simulink model "schemat_macierze"  (R2015a)
settings: Solver=ode45  StartTime=0.0  StopTime=4000  MaxStep=400  RelTol=1e-3
values from neighbouring files (symbols this model uses):
  A = [cpf*Cvp cpf*(Kp+K2)]    [mini_projekt_6b_baza.m]    (also in symulacje_bez_simulinka.m = [-(cpf + K1 + Kp)/Cvw, Kp/Cvw; Kp/Cvp, -(Kp+K2)/Cvp])
  B = [K1*Cvp K1*(Kp+K2)+(Kp*K2)]    [mini_projekt_6b_baza.m]    (also in symulacje_bez_simulinka.m = [cpf/Cvw, K1/Cvw;0,  K2/Cvp])
  C = [cpf*Kp]    [mini_projekt_6b_baza.m]    (also in symulacje_bez_simulinka.m = [1, 0; 0, 1])
  D = [(K2*Cvw) K2*(cpf+K1+Kp)+(Kp*K1)]    [mini_projekt_6b_baza.m]    (also in symulacje_bez_simulinka.m = [0, 0; 0, 0])
  dTkz = 0    [mini_projekt_6b_baza.m]    (also in symulacje_bez_simulinka.m = 2)
  dTzew = 0    [mini_projekt_6b_baza.m]    (also in symulacje_bez_simulinka.m = 2)
  t0 = 5000    [mini_projekt_6b_baza.m]    (also in symulacje_bez_simulinka.m)
  Tkzo = Tkzn    (= 35)    [mini_projekt_6b_baza.m]
  Tpo1 = M*(Kp*Twewo1+K2*Tzewo)    [mini_projekt_6b_baza.m]
  Twewo1 = (cpf*Tkzo+K1*Tzewo+Kp*K2*M*Tzewo)/(cpf+K1+Kp-M*Kp^2)    [mini_projekt_6b_baza.m]
  Tzewo = Tzewn    (= -20)    [mini_projekt_6b_baza.m]
settings Model: Creator=LAB320-1552  LastModifiedBy=apuch
settings DebuggingCC: UnderspecifiedInitializationDetection=Classic  MergeDetectMultiDrivingBlocksExec=none  SolverPrmCheckMsg=warning  StateNameClashWarn=warning

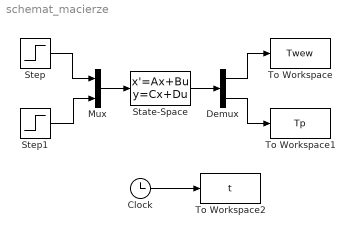
== system schemat_macierze ==
  Clock : Clock
  Demux : Demux  Outputs=2
  Mux : Mux  Inputs=2
  State-Space : StateSpace  A=A  B=B  C=C  D=D  X0=[Twewo1;Tpo1]
  Step : Step  Time=t0  Before=Tkzo  After=Tkzo+dTkz  SampleTime=0
  Step1 : Step  Time=t0  Before=Tzewo  After=Tzewo+dTzew  SampleTime=0
  To Workspace : ToWorkspace  VariableName=Twew  SampleTime=-1
  To Workspace1 : ToWorkspace  VariableName=Tp  SampleTime=-1
  To Workspace2 : ToWorkspace  VariableName=t  SampleTime=-1
  wires:
  Step/1 -> Mux/1
  Step1/1 -> Mux/2
  Mux/1 -> State-Space/1
  State-Space/1 -> Demux/1
  Demux/1 -> To Workspace/1
  Demux/2 -> To Workspace1/1
  Clock/1 -> To Workspace2/1
